simulink model "ControladoresPIDv9_26_04_2026"  (R2025b)
settings: Solver=ode5  StartTime=0.0  StopTime=10  FixedStep=0.0001  RelTol=1e-3
values from neighbouring files (symbols this model uses):
  Bm = 0.008    [definirParametros.m]    (also in definirParametrosMotorElectroCraftDP300.m; definirParametrosMotorElectroCraftDPP728V120.m = Jm/tm; definirParametrosMotorElectroCraftDPP728V120_Optimizador.m = Jm/tm; definirParametrosMotorElectroCraftDPP728V120_v2.m = Jm/tm)
  dm = 0.3    [definirParametros.m]    (also in definirParametrosMotorElectroCraftDP300.m; definirParametrosMotorElectroCraftDPP728V120.m; definirParametrosMotorElectroCraftDPP728V120_Optimizador.m = 0.550061; definirParametrosMotorElectroCraftDPP728V120_v2.m = 0.550061)
  dmc = 0.5    [definirParametros.m]    (also in definirParametrosMotorElectroCraftDP300.m; definirParametrosMotorElectroCraftDPP728V120.m; definirParametrosMotorElectroCraftDPP728V120_Optimizador.m = 1.06911; definirParametrosMotorElectroCraftDPP728V120_v2.m = 1.06911)
  g = 9.8    [definirParametros.m]    (also in definirParametrosMotorElectroCraftDP300.m; definirParametrosMotorElectroCraftDPP728V120.m; definirParametrosMotorElectroCraftDPP728V120_Optimizador.m; definirParametrosMotorElectroCraftDPP728V120_v2.m)
  Jm = gramsCM2ToKgMeters2(12358.5)    [definirParametrosMotorElectroCraftDPP728V120.m]    (also in definirParametrosMotorElectroCraftDPP728V120_Optimizador.m; definirParametrosMotorElectroCraftDPP728V120_v2.m; definirParametrosMotorElectroCraftDPP728V120_v3.m; definirParametrosMotorElectroCraftRP34M221V90.m = gramsCM2ToKgMeters2(2718.9))
  Kb = 0.6    [definirParametros.m]    (also in definirParametrosMotorElectroCraftDP300.m = VoltagePerKRPMToVoltagePerHertz(12.3); definirParametrosMotorElectroCraftDPP728V120.m = VoltagePerKRPMToVoltagePerRadS(64.9); definirParametrosMotorElectroCraftDPP728V120_Optimizador.m = VoltagePerKRPMToVoltagePerRadS(64.9); definirParametrosMotorElectroCraftDPP728V120_v2.m = VoltagePerKRPMToVoltagePerRadS(64.9))
  Kt = 0.7274    [definirParametros.m]    (also in definirParametrosMotorElectroCraftDP300.m = newtonCMToNewtonM(11.722); definirParametrosMotorElectroCraftDPP728V120.m = newtonCMToNewtonM(62); definirParametrosMotorElectroCraftDPP728V120_Optimizador.m = newtonCMToNewtonM(62); definirParametrosMotorElectroCraftDPP728V120_v2.m = newtonCMToNewtonM(62))
  Lm = 4.3/1000    (= 0.0043)    [definirParametrosMotorElectroCraftDPP728V120.m]    (also in definirParametrosMotorElectroCraftDPP728V120_Optimizador.m; definirParametrosMotorElectroCraftDPP728V120_v2.m; definirParametrosMotorElectroCraftDPP728V120_v3.m; definirParametrosMotorElectroCraftDPP728V60.m = 0.0015)
  Mc = 200    [definirParametros.m]    (also in definirParametrosMotorElectroCraftDP300.m; definirParametrosMotorElectroCraftDPP728V120.m; definirParametrosMotorElectroCraftDPP728V120_Optimizador.m = 144.6; definirParametrosMotorElectroCraftDPP728V120_v2.m = 144.6)
  Mm = 100    [definirParametros.m]    (also in definirParametrosMotorElectroCraftDP300.m; definirParametrosMotorElectroCraftDPP728V120.m; definirParametrosMotorElectroCraftDPP728V120_Optimizador.m = 18.911; definirParametrosMotorElectroCraftDPP728V120_v2.m = 18.911)
  pPosicion = znHallarKPOfPController(KCriticaPosicion)    [HallarValoresPID.m]
  relacionEngranajes = 100.0/1    (= 100)    [definirParametros.m]    (also in definirParametrosMotorElectroCraftDP300.m = 1; definirParametrosMotorElectroCraftDPP728V120.m; definirParametrosMotorElectroCraftDPP728V120_Optimizador.m; definirParametrosMotorElectroCraftDPP728V120_v2.m)
  Rm = 1.55    [definirParametrosMotorElectroCraftDPP728V120.m]    (also in definirParametrosMotorElectroCraftDPP728V120_Optimizador.m; definirParametrosMotorElectroCraftDPP728V120_v2.m; definirParametrosMotorElectroCraftDPP728V120_v3.m; definirParametrosMotorElectroCraftDPP728V60.m = 0.72)
libraries: simulink x12, slpidlib x2
settings Model: Creator=rghuertaspaiva  LastModifiedBy=User
settings SolverCC: AlgebraicLoopSolver=TrustRegion
settings DebuggingCC: UnconnectedInputMsg=warning  UnconnectedOutputMsg=warning  UnconnectedLineMsg=warning
settings ModelReferenceCC: EnableRefExpFcnMdlSchedulingChecks=on
settings RTWCC: GPUComputeCapability=3.5

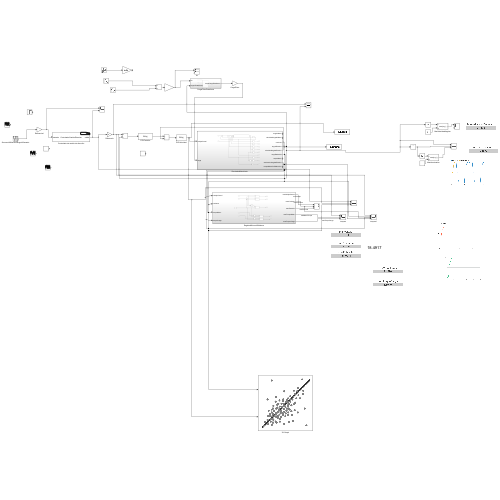
[thumbnail: Simulink's stored preview of the top-level diagram]
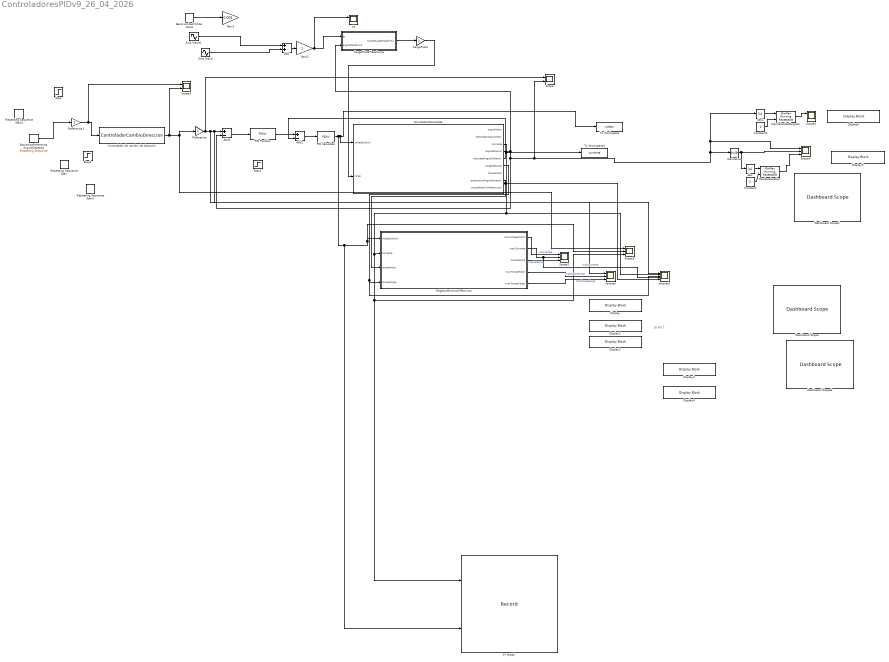
== system ControladoresPIDv9_26_04_2026 ==
  note: 18.4917
  Abs : Abs  SaturateOnIntegerOverflow=off
  Abs1 : Abs  SaturateOnIntegerOverflow=off
  Add : Sum
  Add1 : Sum  Inputs=+-
  Add2 : Sum  Inputs=+-
  Band-Limited White Noise : simulink/Sources/Band-Limited White Noise  Cov=[.12]  Ts=0.05  seed=[23341]
  CargaPiloto : Gain
  CargaPilotoPlataforma : Subsystem
  Constant : Constant  Value=0
  Constant1 : Constant  Value=0
  Controlador de cambio de dirección : S-Function  InitFcn=try, set_param(gcb,'FunctionName','ControladorCambioDireccion'), end  FunctionName=ControladorCambioDireccion  SFunctionModules=ControladorCambioDireccion_wrapper  SFunctionDeploymentMode=off  EnableBusSupport=off  mask(S-Function Builder){}
      mask help: Simulink:masks:SFunctionBuilder_MD
      mask init:
      | val = [[.9  0.75 0.75 1 1 .9 .9 1]',[1 1 0.75 0.75 .9 .9 1 .9]'];try , sys = get_param(gcb,'SfunBuilderFcnName');if isempty(sys), sys = get_param(gcb,'FunctionName'); end,catch, sys = get_param(gcb,'FunctionName'); end
      settings: CopyFcn=set_param(gcbh,'LinkStatus','none')  PreSaveFcn=try, set_param(gcb,'FunctionName','ControladorCambioDireccion'), end  OpenFcn=sfunctionwizard(gcbh)
      mask Display: plot(val(:,1),val(:,2)),disp(sys), port_label('input',1,'entrada'), port_label('output',1,'salida')
  Dashboard Scope : DashboardScope  FontColor=[0.0, 0.0, 0.0]
  Dashboard Scope1 : DashboardScope  FontColor=[0.0, 0.0, 0.0]
  Dashboard Scope3 : DashboardScope  FontColor=[0.0, 0.0, 0.0]
  Derivative : Derivative
  Display{,1..6} (7 alike) : DisplayBlock  Transparency=1  GridColor=[0.502, 0.502, 0.502]
  Gain1 : Gain  Gain=0.005
  Gain2 : Gain
  MaxAcceleration : simulink/Math Operations/MinMax Running Resettable  Function=max  vinit=0.0
  MaxVelocidadAngular : simulink/Math Operations/MinMax Running Resettable  Function=max  vinit=0.0
  PID Posiciǿn : slpidlib/PID Controller  Controller=PID  Form=Parallel  TimeDomain=Continuous-time  UseExternalTs=off  SampleTime=-1  IntegratorMethod=Forward Euler  FilterMethod=Forward Euler  ControllerParametersSource=internal  P=pPosicion  I=0  UseKiTs=off  D=0  UseExternalDerivativeSource=off  N=83.8286578398202  UseFilter=on  TunerSelectOption=Transfer Function Based (PID Tuner App)  InitialConditionSource=internal  InitialConditionForIntegrator=0  InitialConditionForFilter=0  DifferentiatorICPrevScaledInput=0  ExternalReset=none  TrackingMode=off  Kt=1  LimitOutput=off  SatLimitsSource=internal  UpperSaturationLimit=inf  LowerSaturationLimit=-inf  LinearizeAsGain=on  AntiWindupMode=none  Kb=1  LimitIntegrator=off  UpperIntegratorSaturationLimit=inf  LowerIntegratorSaturationLimit=-inf  POutMin=[]  POutMax=[]  IOutMin=[]  IOutMax=[]  DOutMin=[]  DOutMax=[]  NOutMin=[]  NOutMax=[]  SumOutMin=[]  SumOutMax=[]  SaturationOutMin=[]  SaturationOutMax=[]  PParamMin=[]  PParamMax=[]  IParamMin=[]  IParamMax=[]  DParamMin=[]  DParamMax=[]  NParamMin=[]  NParamMax=[]  KbParamMin=[]  KbParamMax=[]  KtParamMin=[]  KtParamMax=[]  KbOutMin=[]  KbOutMax=[]  KtOutMin=[]  KtOutMax=[]  IntegratorOutMin=[]  IntegratorOutMax=[]  FilterOutMin=[]  FilterOutMax=[]  SumI1OutMin=[]  SumI1OutMax=[]  SumI2OutMin=[]  SumI2OutMax=[]  SumI3OutMin=[]  SumI3OutMax=[]  SumI4OutMin=[]  SumI4OutMax=[]  SumDOutMin=[]  SumDOutMax=[]  DifferentiatorOutMin=[]  DifferentiatorOutMax=[]  FilterDiffOutCoefMin=[]  FilterDiffOutCoefMax=[]  ReciprocalOutMin=[]  ReciprocalOutMax=[]  SumDenOutMin=[]  SumDenOutMax=[]  SumNumOutMin=[]  SumNumOutMax=[]  DivideOutMin=[]  DivideOutMax=[]  UdiffTsProdOutMin=[]  UdiffTsProdOutMax=[]  NTsProdOutMin=[]  NTsProdOutMax=[]  UintegralTsProdOutMin=[]  UintegralTsProdOutMax=[]  UngainTsProdOutMin=[]  UngainTsProdOutMax=[]  ClampingZeroOutDataTypeStr=Inherit: Inherit via back propagation  ClampingZeroOutMin=[]  ClampingZeroOutMax=[]  FilterDenConstantOutDataTypeStr=Inherit: Inherit via back propagation  FilterDenConstantOutMin=[]  FilterDenConstantOutMax=[]  PCopyOutDataTypeStr=Inherit: Inherit via back propagation  PCopyOutMin=[]  PCopyOutMax=[]  NCopyOutDataTypeStr=Inherit: Inherit via back propagation  NCopyOutMin=[]  NCopyOutMax=[]  IntegratorContinuousStateAttributes=''  IntegratorStateMustResolveToSignalObject=off  IntegratorRTWStateStorageClass=Auto  FilterContinuousStateAttributes=''  FilterStateMustResolveToSignalObject=off  FilterRTWStateStorageClass=Auto  ParallelPVariant=InternalParameters  IdealPVariant=Disabled  IVariant=InternalParameters  DVariant=InternalParameters  IntegratorVariant=Continuous  SatVariant=Disabled  AWVariant=Passthrough  PCopyVariant=Disabled  TRVariant=Disabled  FdbkBlocksVariant=Forward  IdealPFdbkVariant=Disabled  SatFdbkVariant=Disabled  DerivativeFilterVariant=ContFilter  NVariant=InternalParameters  NCopyVariant=Disabled  FilterICVariant=InternalICsFilter  IntegratorICVariant=InternalICs  ExternalResetVariant=Disabled  TRSumVariant=Passthrough  SumFdbkVariant=Disabled  SumVariant=Sum_PID  TsampFilterVariant=InternalTs  TsampNgainVariant=Passthrough  TsampIntegralVariant=Disabled_SignalSpec  ExternalSaturationOutDataTypeStr=Inherit: Same as second input  DerivativeSourceVariant=ErrorSignal  PreIntVariant=InternalPreInt
  PID Velocidad : slpidlib/PID Controller  Controller=PID  Form=Parallel  TimeDomain=Continuous-time  UseExternalTs=off  SampleTime=-1  IntegratorMethod=Forward Euler  FilterMethod=Forward Euler  ControllerParametersSource=internal  P=3840  I=0  UseKiTs=off  D=0  UseExternalDerivativeSource=off  N=100  UseFilter=on  TunerSelectOption=Transfer Function Based (PID Tuner App)  InitialConditionSource=internal  InitialConditionForIntegrator=0  InitialConditionForFilter=0  DifferentiatorICPrevScaledInput=0  ExternalReset=none  TrackingMode=off  Kt=1  LimitOutput=off  SatLimitsSource=internal  UpperSaturationLimit=inf  LowerSaturationLimit=-inf  LinearizeAsGain=on  AntiWindupMode=none  Kb=1  LimitIntegrator=off  UpperIntegratorSaturationLimit=inf  LowerIntegratorSaturationLimit=-inf  POutMin=[]  POutMax=[]  IOutMin=[]  IOutMax=[]  DOutMin=[]  DOutMax=[]  NOutMin=[]  NOutMax=[]  SumOutMin=[]  SumOutMax=[]  SaturationOutMin=[]  SaturationOutMax=[]  PParamMin=[]  PParamMax=[]  IParamMin=[]  IParamMax=[]  DParamMin=[]  DParamMax=[]  NParamMin=[]  NParamMax=[]  KbParamMin=[]  KbParamMax=[]  KtParamMin=[]  KtParamMax=[]  KbOutMin=[]  KbOutMax=[]  KtOutMin=[]  KtOutMax=[]  IntegratorOutMin=[]  IntegratorOutMax=[]  FilterOutMin=[]  FilterOutMax=[]  SumI1OutMin=[]  SumI1OutMax=[]  SumI2OutMin=[]  SumI2OutMax=[]  SumI3OutMin=[]  SumI3OutMax=[]  SumI4OutMin=[]  SumI4OutMax=[]  SumDOutMin=[]  SumDOutMax=[]  DifferentiatorOutMin=[]  DifferentiatorOutMax=[]  FilterDiffOutCoefMin=[]  FilterDiffOutCoefMax=[]  ReciprocalOutMin=[]  ReciprocalOutMax=[]  SumDenOutMin=[]  SumDenOutMax=[]  SumNumOutMin=[]  SumNumOutMax=[]  DivideOutMin=[]  DivideOutMax=[]  UdiffTsProdOutMin=[]  UdiffTsProdOutMax=[]  NTsProdOutMin=[]  NTsProdOutMax=[]  UintegralTsProdOutMin=[]  UintegralTsProdOutMax=[]  UngainTsProdOutMin=[]  UngainTsProdOutMax=[]  ClampingZeroOutDataTypeStr=Inherit: Inherit via back propagation  ClampingZeroOutMin=[]  ClampingZeroOutMax=[]  FilterDenConstantOutDataTypeStr=Inherit: Inherit via back propagation  FilterDenConstantOutMin=[]  FilterDenConstantOutMax=[]  PCopyOutDataTypeStr=Inherit: Inherit via back propagation  PCopyOutMin=[]  PCopyOutMax=[]  NCopyOutDataTypeStr=Inherit: Inherit via back propagation  NCopyOutMin=[]  NCopyOutMax=[]  IntegratorContinuousStateAttributes=''  IntegratorStateMustResolveToSignalObject=off  IntegratorRTWStateStorageClass=Auto  FilterContinuousStateAttributes=''  FilterStateMustResolveToSignalObject=off  FilterRTWStateStorageClass=Auto  ParallelPVariant=InternalParameters  IdealPVariant=Disabled  IVariant=InternalParameters  DVariant=InternalParameters  IntegratorVariant=Continuous  SatVariant=Disabled  AWVariant=Passthrough  PCopyVariant=Disabled  TRVariant=Disabled  FdbkBlocksVariant=Forward  IdealPFdbkVariant=Disabled  SatFdbkVariant=Disabled  DerivativeFilterVariant=ContFilter  NVariant=InternalParameters  NCopyVariant=Disabled  FilterICVariant=InternalICsFilter  IntegratorICVariant=InternalICs  ExternalResetVariant=Disabled  TRSumVariant=Passthrough  SumFdbkVariant=Disabled  SumVariant=Sum_PID  TsampFilterVariant=InternalTs  TsampNgainVariant=Passthrough  TsampIntegralVariant=Disabled_SignalSpec  ExternalSaturationOutDataTypeStr=Inherit: Same as second input  DerivativeSourceVariant=ErrorSignal  PreIntVariant=InternalPreInt
  Referencia : Gain
  Referencia1 : Gain
  RegistroMínimosYMáximos : Subsystem
  Repeating Sequence Stair : simulink/Sources/Repeating Sequence Stair  OutValues="[0 1 1 0 0 -1 -1  0 0  1 1 -1 -1 1 1]"  tsamp=1  OutMin=[]  OutMax=[]  OutDataTypeStr=double  OutputDataTypeScalingMode=double  OutDataType=fixdt(0,8)  ConRadixGroup=Best Precision: Vector-wise  OutScaling=2^-12
  Repeating Sequence Stair1 : simulink/Sources/Repeating Sequence Stair  OutValues="[0 1 -1 1 -1 1  -1 ]"  tsamp=1  OutMin=[]  OutMax=[]  OutDataTypeStr=double  OutputDataTypeScalingMode=double  OutDataType=fixdt(0,8)  ConRadixGroup=Best Precision: Vector-wise  OutScaling=2^-12
  Repeating Sequence Stair2 : simulink/Sources/Repeating Sequence Stair  OutValues="[0 1 1 -1 -1 1 1  -1 -1 ]"  tsamp=1  OutMin=[]  OutMax=[]  OutDataTypeStr=double  OutputDataTypeScalingMode=double  OutDataType=fixdt(0,8)  ConRadixGroup=Best Precision: Vector-wise  OutScaling=2^-12
  Scope : Scope  NumInputPorts=2
      settings: ActiveDisplayYMinimum=-0.21832978644162951  ActiveDisplayYMaximum=0.32465698973435358
  Scope{1..2,4..5} (4 alike) : Scope  NumInputPorts=3
      Scope1 settings: ActiveDisplayYMinimum=-3746.48788  ActiveDisplayYMaximum=33718.39095
      Scope2 settings: ActiveDisplayYMinimum=-82.074709415775956  ActiveDisplayYMaximum=143.37677856471112
      Scope4 settings: ActiveDisplayYMinimum=-16.172410843498408  ActiveDisplayYMaximum=28.3036012317205  DataLoggingVariableName=ScopeData3
      Scope5 settings: ActiveDisplayYMinimum=-12.516355883973082  ActiveDisplayYMaximum=24.074169319183135  DataLoggingVariableName=ScopeData5
  Scope3 : Scope  NumInputPorts=2
      settings: ActiveDisplayYMinimum=-2.5673172788401826  ActiveDisplayYMaximum=1.8523832517968768  DataLoggingVariableName=ScopeData2
  SecuenciaReferenciaAnguloDeseado : simulink/Sources/Repeating Sequence  rep_seq_t=secuencia_tiempo  rep_seq_y=secuencia_valores
  SimuladorMotocicleta : Subsystem
  Sine Wave : Sin  Amplitude=0.015  Frequency=2*pi/4  SampleTime=0
  Sine Wave1 : Sin  Amplitude=0.005  Frequency=10*2*pi  SampleTime=0
  Step : Step  After=deg2rad(7)  SampleTime=0
  Step1 : Step  After=deg2rad(30)  SampleTime=0
  Step2 : Step  After=deg2rad(30)  SampleTime=0
  To Workspace : ToWorkspace  VariableName=voltaje  SaveFormat=Timeseries  SampleTime=-1
  To Workspace1 : ToWorkspace  VariableName=corriente  SaveFormat=Timeseries  SampleTime=-1
  XY Graph : Record  NumPorts=2.0  FileSettingsInternal="{\"entries\":[{\"content\":{\"excelSettings\":{\"content\":{},\"type\":\"Streamout.ExcelSettings\"},\"parquetSettings\":{\"content\":{},\"type\":\"Streamout.ParquetSettings\"}},\"type\":\"Streamout.FileSettingStorage\",\"uuid\":\"\"}],\"packageUris\":[\"http:\\/\\/schema.mathworks.com\\/mf0\\/streamout_blocks\\/R2020a\"],\"version\":\"1.0\"}"  FrameSettings=[0, 0]  Layout=[1 1]  SignalsInternal="{\"entries\":[{\"content\":{\"signals\":[{\"content\":{\"blockPath\":[],\"dimensions\":[1],\"domain\":\"\",\"lineColor\":\"#fe330a\",\"lineWidth\":2,\"plots\":[ 1 ],\"port\":1,\"sid\":[\"\"],\"signalID\":1,\"signalName\":\"SimuladorMotocicleta:3\"},\"type\":\"RecordBlkView.Signal\",\"uuid\":\"\"},{\"content\":{\"blockPath\":[],\"dimensions\":[1],\"domain\":\"\",\"lineColor\":\"#139fff\",\"plots\":[ 1 ],\"port\":2,\"sid\":[\"\"],\"signalID\":2,\"signalName\":\"PID Velocidad\"},\"type\":\"RecordBlkView.Signal\",\"uuid\":\"\"}]},\"type\":\"RecordBlkView.InputSignals\",\"uuid\":\"\"}],\"packageUris\":[\"http:\\/\\/schema.mathworks.com\\/mf0\\/streamout_blocks\\/R2020a\"],\"version\":\"1.0\"}"  VisualizationBindings="{\"xyplotplugin\":{\"info\":[{\"series\":[{\"bindingParametersList\":[{\"parameter\":\"X-Axis\",\"signalID\":1,\"signalName\":\"SimuladorMotocicleta:3\"},{\"parameter\":\"Y-Axis\",\"signalID\":2,\"signalName\":\"PID Velocidad\"}],\"seriesID\":0}],\"subplotID\":1}]}}"  CompatibilityTag=XY  st=-1
  dc : Scope  NumInputPorts=2
      settings: ActiveDisplayYMinimum=-0.66544385540690021  ActiveDisplayYMaximum=0.32129499518952043  DataLoggingVariableName=ScopeData4
  torques : Scope  NumInputPorts=3
      settings: ActiveDisplayYMinimum=-1.6922292408807111  ActiveDisplayYMaximum=8.3664080257188083
  torques1 : Scope  NumInputPorts=5
      settings: ActiveDisplayYMinimum=-14.71989952294008  ActiveDisplayYMaximum=14.945739054536634  DataLoggingVariableName=ScopeData2
  wires:
  Sine Wave/1 -> Add/2
  CargaPilotoPlataforma/1(torqueCargaPlataforma) -> CargaPiloto/1
  PID Velocidad/1 -> XY Graph/2, Scope2/2, RegistroMínimosYMáximos/1(voltajeControl), SimuladorMotocicleta/1(voltajeControl), To Workspace/1
  Add1/1 -> PID Velocidad/1
  SimuladorMotocicleta/5(velocidadAngularExterior) -> Add1/2
  Referencia/1 -> Scope/1, torques/1, torques1/1, Add2/1
  Add2/1 -> PID Posiciǿn/1
  SimuladorMotocicleta/3(corriente) -> To Workspace1/1, torques1/2, XY Graph/1, Scope2/3, RegistroMínimosYMáximos/2(corriente)
  RegistroMínimosYMáximos/1(maxVoltajeControl) -> Scope1/1  "maxVoltaje"
  RegistroMínimosYMáximos/2(maxCorriente) -> torques1/4, Scope1/2  "maxCorriente"
  PID Posiciǿn/1 -> Add1/1
  RegistroMínimosYMáximos/3(maxPotencia) -> Scope1/3  "maxPotencia"
  Controlador de cambio de dirección/1 -> Scope2/1, Referencia/1, Scope3/2
  RegistroMínimosYMáximos/4(maxTorqueMotor) -> torques/2  "maxMotorTorque"
  RegistroMínimosYMáximos/5(maxTorqueCarga) -> torques/3  "maxTorqueCarga"
  SimuladorMotocicleta/8(aceleracionAngularExterior) -> torques1/5, RegistroMínimosYMáximos/3(torqueMotor)
  SimuladorMotocicleta/6(cargaReducida) -> torques1/3, RegistroMínimosYMáximos/4(torqueCarga)
  Derivative/1 -> Abs/1, Scope4/2
  SimuladorMotocicleta/4(anguloExterior) -> Add2/2, Abs1/1, Scope4/1, Derivative/1, Scope/2, CargaPilotoPlataforma/2(anguloPlataforma)
  MaxAcceleration/1 -> Scope4/3
  Abs/1 -> MaxAcceleration/1
  Constant/1 -> MaxAcceleration/2
  Gain2/1 -> dc/1, CargaPilotoPlataforma/1(dc)
  Add/1 -> Gain2/1
  Abs1/1 -> MaxVelocidadAngular/1
  Constant1/1 -> MaxVelocidadAngular/2
  MaxVelocidadAngular/1 -> Scope5/1
  Band-Limited White Noise/1 -> Gain1/1
  Sine Wave1/1 -> Add/1
  Referencia1/1 -> Scope3/1, Controlador de cambio de dirección/1
  SecuenciaReferenciaAnguloDeseado/1 -> Referencia1/1
  CargaPiloto/1 -> SimuladorMotocicleta/2(carga)

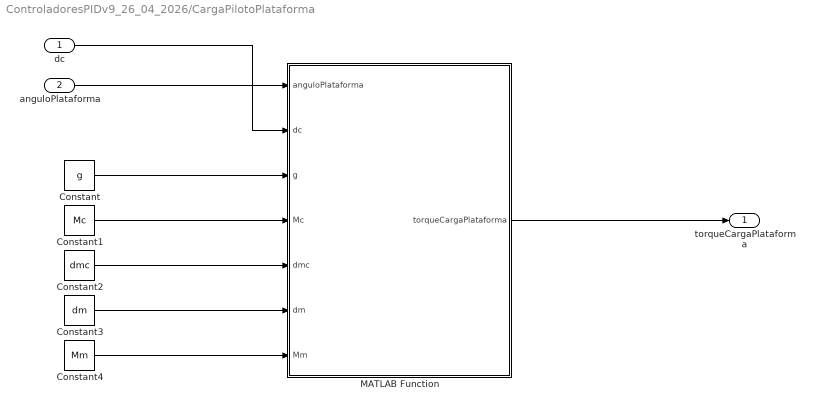
== system ControladoresPIDv9_26_04_2026/CargaPilotoPlataforma ==
  dc : Inport
  anguloPlataforma : Inport  Port=2
  Constant : Constant  Value=g
  Constant1 : Constant  Value=Mc
  Constant2 : Constant  Value=dmc
  Constant3 : Constant  Value=dm
  Constant4 : Constant  Value=Mm
  MATLAB Function : MATLAB Function  TreatAsAtomicUnit=on
  torqueCargaPlataforma : Outport
  wires:
  dc/1 -> MATLAB Function/2(dc)
  anguloPlataforma/1 -> MATLAB Function/1(anguloPlataforma)
  Constant/1 -> MATLAB Function/3(g)
  Constant1/1 -> MATLAB Function/4(Mc)
  Constant2/1 -> MATLAB Function/5(dmc)
  Constant3/1 -> MATLAB Function/6(dm)
  Constant4/1 -> MATLAB Function/7(Mm)
  MATLAB Function/1(torqueCargaPlataforma) -> torqueCargaPlataforma/1

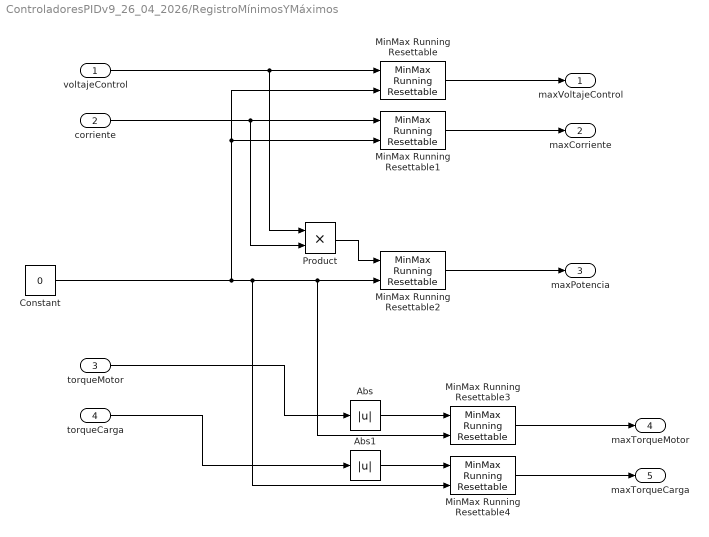
== system ControladoresPIDv9_26_04_2026/RegistroMínimosYMáximos ==
  voltajeControl : Inport
  corriente : Inport  Port=2
  torqueMotor : Inport  Port=3
  torqueCarga : Inport  Port=4
  Abs : Abs  SaturateOnIntegerOverflow=off
  Abs1 : Abs  SaturateOnIntegerOverflow=off
  Constant : Constant  Value=0
  MinMax Running Resettable{,1..4} (5 alike) : simulink/Math Operations/MinMax Running Resettable  Function=max  vinit=0.0
  Product : Product
  maxVoltajeControl : Outport
  maxCorriente : Outport  Port=2
  maxPotencia : Outport  Port=3
  maxTorqueMotor : Outport  Port=4
  maxTorqueCarga : Outport  Port=5
  wires:
  voltajeControl/1 -> Product/1, MinMax Running Resettable/1
  corriente/1 -> Product/2, MinMax Running Resettable1/1
  Constant/1 -> MinMax Running Resettable1/2, MinMax Running Resettable/2, MinMax Running Resettable4/2, MinMax Running Resettable3/2, MinMax Running Resettable2/2
  MinMax Running Resettable/1 -> maxVoltajeControl/1
  MinMax Running Resettable1/1 -> maxCorriente/1
  Product/1 -> MinMax Running Resettable2/1
  MinMax Running Resettable2/1 -> maxPotencia/1
  MinMax Running Resettable4/1 -> maxTorqueCarga/1
  MinMax Running Resettable3/1 -> maxTorqueMotor/1
  torqueMotor/1 -> Abs/1
  torqueCarga/1 -> Abs1/1
  Abs/1 -> MinMax Running Resettable3/1
  Abs1/1 -> MinMax Running Resettable4/1

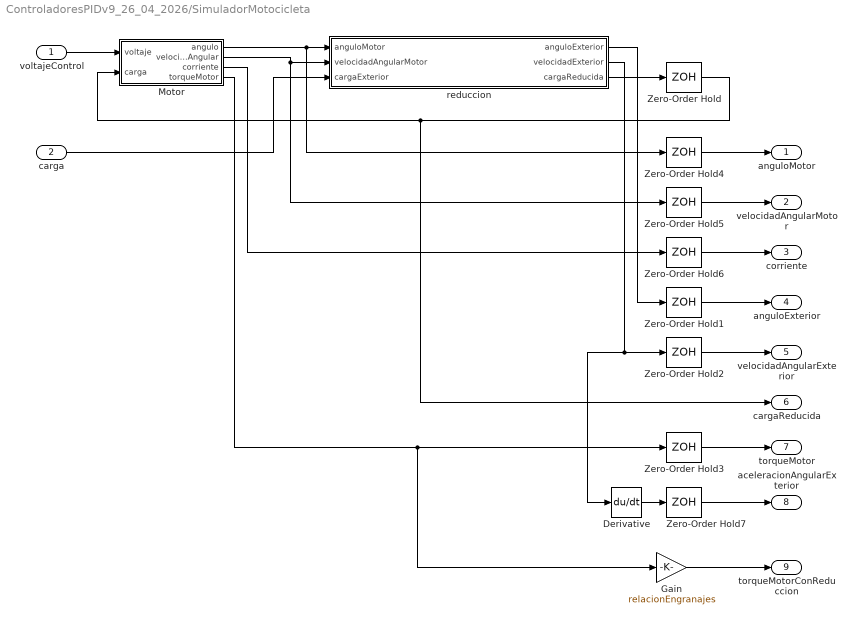
== system ControladoresPIDv9_26_04_2026/SimuladorMotocicleta ==
  voltajeControl : Inport
  carga : Inport  Port=2
  Derivative : Derivative
  Gain : Gain  Gain=relacionEngranajes
  Motor : Subsystem
  Zero-Order Hold{,1..7} (8 alike) : ZeroOrderHold  SampleTime=-1
  reduccion : Subsystem
  anguloMotor : Outport
  velocidadAngularMotor : Outport  Port=2
  corriente : Outport  Port=3
  anguloExterior : Outport  Port=4
  velocidadAngularExterior : Outport  Port=5
  cargaReducida : Outport  Port=6
  torqueMotor : Outport  Port=7
  aceleracionAngularExterior : Outport  Port=8
  torqueMotorConReduccion : Outport  Port=9
  wires:
  Gain/1 -> torqueMotorConReduccion/1
  Motor/4(torqueMotor) -> Gain/1, Zero-Order Hold3/1
  Motor/2(velocidadAngular) -> Zero-Order Hold5/1, reduccion/2(velocidadAngularMotor)
  Derivative/1 -> Zero-Order Hold7/1
  Motor/1(angulo) -> Zero-Order Hold4/1, reduccion/1(anguloMotor)
  Motor/3(corriente) -> Zero-Order Hold6/1
  Zero-Order Hold6/1 -> corriente/1
  Zero-Order Hold5/1 -> velocidadAngularMotor/1
  reduccion/3(cargaReducida) -> Zero-Order Hold/1
  Zero-Order Hold3/1 -> torqueMotor/1
  Zero-Order Hold2/1 -> velocidadAngularExterior/1
  Zero-Order Hold1/1 -> anguloExterior/1
  Zero-Order Hold4/1 -> anguloMotor/1
  reduccion/2(velocidadExterior) -> Derivative/1, Zero-Order Hold2/1
  Zero-Order Hold7/1 -> aceleracionAngularExterior/1
  Zero-Order Hold/1 -> cargaReducida/1, Motor/2(carga)
  carga/1 -> reduccion/3(cargaExterior)
  reduccion/1(anguloExterior) -> Zero-Order Hold1/1
  voltajeControl/1 -> Motor/1(voltaje)

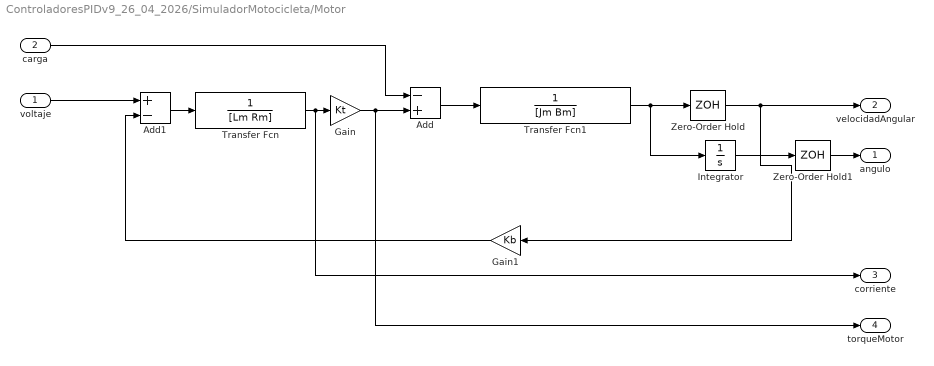
== system ControladoresPIDv9_26_04_2026/SimuladorMotocicleta/Motor ==
  voltaje : Inport
  carga : Inport  Port=2
  Add : Sum  Inputs=-+
  Add1 : Sum  Inputs=+-
  Gain : Gain  Gain=Kt
  Gain1 : Gain  Gain=Kb
  Integrator : Integrator
  Transfer Fcn : TransferFcn  Denominator=[Lm Rm]
  Transfer Fcn1 : TransferFcn  Denominator=[Jm Bm]
  Zero-Order Hold : ZeroOrderHold  SampleTime=-1
  Zero-Order Hold1 : ZeroOrderHold  SampleTime=-1
  angulo : Outport
  velocidadAngular : Outport  Port=2
  corriente : Outport  Port=3
  torqueMotor : Outport  Port=4
  wires:
  Gain/1 -> torqueMotor/1, Add/2
  Add/1 -> Transfer Fcn1/1
  Transfer Fcn/1 -> corriente/1, Gain/1
  Transfer Fcn1/1 -> Integrator/1, Zero-Order Hold/1
  Zero-Order Hold/1 -> Gain1/1, velocidadAngular/1
  Integrator/1 -> Zero-Order Hold1/1
  voltaje/1 -> Add1/1
  Add1/1 -> Transfer Fcn/1
  Gain1/1 -> Add1/2
  carga/1 -> Add/1
  Zero-Order Hold1/1 -> angulo/1

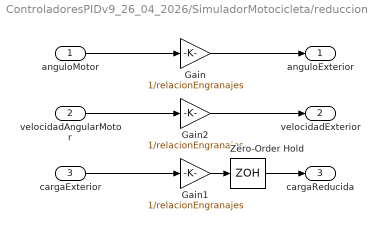
== system ControladoresPIDv9_26_04_2026/SimuladorMotocicleta/reduccion ==
  anguloMotor : Inport
  velocidadAngularMotor : Inport  Port=2
  cargaExterior : Inport  Port=3
  Gain : Gain  Gain=1/relacionEngranajes
  Gain1 : Gain  Gain=1/relacionEngranajes
  Gain2 : Gain  Gain=1/relacionEngranajes
  Zero-Order Hold : ZeroOrderHold  SampleTime=-1
  anguloExterior : Outport
  velocidadExterior : Outport  Port=2
  cargaReducida : Outport  Port=3
  wires:
  anguloMotor/1 -> Gain/1
  Gain/1 -> anguloExterior/1
  cargaExterior/1 -> Gain1/1
  Gain1/1 -> Zero-Order Hold/1
  velocidadAngularMotor/1 -> Gain2/1
  Gain2/1 -> velocidadExterior/1
  Zero-Order Hold/1 -> cargaReducida/1

== matlab function ControladoresPIDv9_26_04_2026/CargaPilotoPlataforma/MATLAB Function ==
  data: anguloPlataforma input; torqueCargaPlataforma output; dc input; g input; Mc input; dmc input; dm input; Mm input
function torqueCargaPlataforma = torquePlataformaPiloto(anguloPlataforma, dc, g, Mc, dmc, dm, Mm)


torqueCargaPlataforma =  g*( dc*Mc*cos(anguloPlataforma) + ...
                             (dmc*Mc + dm*(Mc + Mm))*sin(anguloPlataforma) ...
                           );
